simulink model "feedback_control_simulink"  (R2026a)
settings: Solver=VariableStepAuto
settings Model: Creator=PC-Admin  LastModifiedBy=PC-Admin

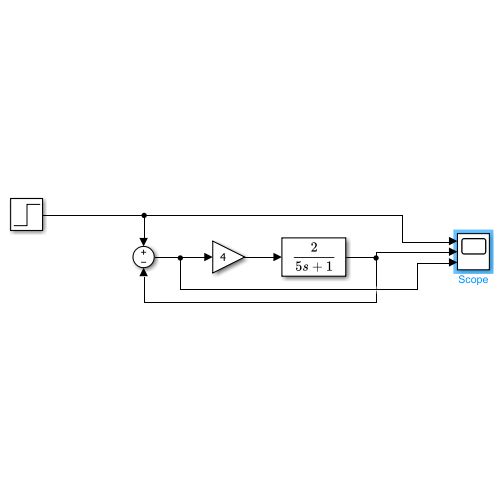
[thumbnail: Simulink's stored preview of the top-level diagram]
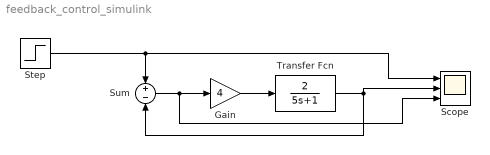
== system feedback_control_simulink ==
  Gain : Gain  Gain=4
  Scope : Scope  NumInputPorts=3
      settings: ActiveDisplayYMinimum=-0.53726629170480966  ActiveDisplayYMaximum=1.5779678427555111
  Step : Step  SampleTime=0
  Sum : Sum  Inputs=+-
  Transfer Fcn : TransferFcn  Numerator=[2]  Denominator=[5 1]
  wires:
  Step/1 -> Scope/1, Sum/1
  Sum/1 -> Scope/3, Gain/1
  Gain/1 -> Transfer Fcn/1
  Transfer Fcn/1 -> Sum/2, Scope/2
